simulink model "test"  (R2022a)
settings: Solver=VariableStepAuto  StartTime=0.0  StopTime=20  MaxStep=0.001  RelTol=1e-3
values from neighbouring files (symbols this model uses):
  SysMat = ss(Lmat)    [config.m]    (also in test_conf.m)
  SysVec = ss(Lvec)    [config.m]    (also in test_conf.m)
settings Model: Creator=Vvlad  LastModifiedBy=Vvlad

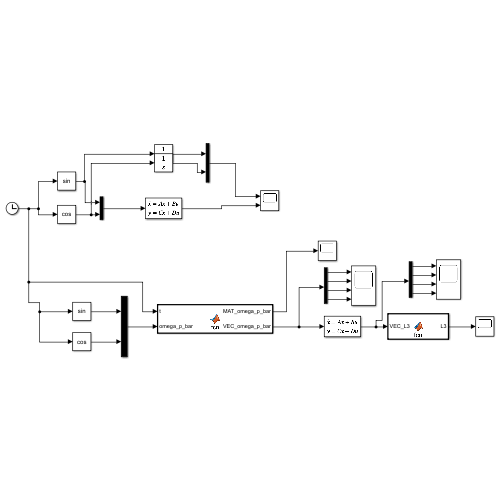
[thumbnail: Simulink's stored preview of the top-level diagram]
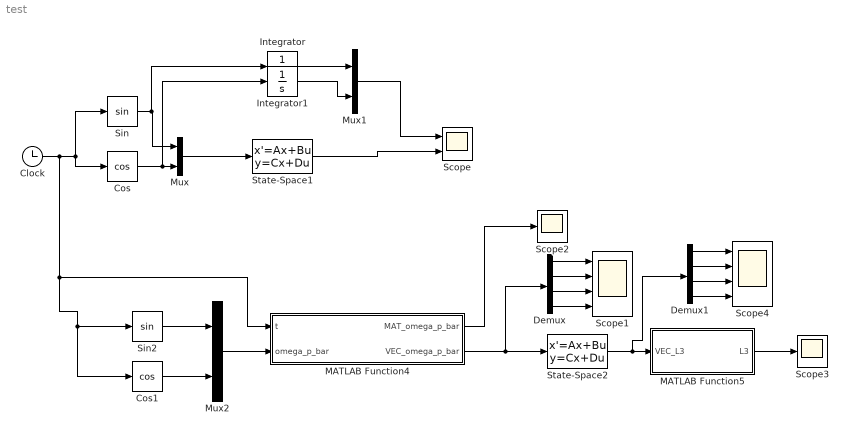
== system test ==
  Clock : Clock
  Cos : Trigonometry  Operator=cos
  Cos1 : Trigonometry  Operator=cos
  Demux : Demux
  Demux1 : Demux
  Integrator : Integrator
  Integrator1 : Integrator
  MATLAB Function4 : MATLAB Function  TreatAsAtomicUnit=on
  MATLAB Function5 : MATLAB Function  TreatAsAtomicUnit=on
  Mux : Mux  Inputs=2
  Mux1 : Mux  Inputs=2
  Mux2 : Mux  Inputs=2
  Scope : Scope  NumInputPorts=2
  Scope1 : Scope  NumInputPorts=4
  Scope2 : Scope
  Scope3 : Scope
  Scope4 : Scope  NumInputPorts=4
  Sin : Trigonometry
  Sin2 : Trigonometry
  State-Space1 : StateSpace  A=SysVec.A  B=SysVec.B  C=SysVec.C  D=SysVec.D  InitialCondition=0
  State-Space2 : StateSpace  A=SysMat.A  B=SysMat.B  C=SysMat.C  D=SysMat.D  InitialCondition=0
  wires:
  Sin/1 -> Integrator/1, Mux/1
  Clock/1 -> MATLAB Function4/1(t), Cos1/1, Sin2/1, Sin/1, Cos/1
  Cos/1 -> Integrator1/1, Mux/2
  Mux/1 -> State-Space1/1
  Integrator1/1 -> Mux1/2
  Integrator/1 -> Mux1/1
  State-Space1/1 -> Scope/2
  Mux1/1 -> Scope/1
  Cos1/1 -> Mux2/2
  Sin2/1 -> Mux2/1
  MATLAB Function4/2(VEC_omega_p_bar) -> Demux/1, State-Space2/1
  Demux/1 -> Scope1/1
  Demux/2 -> Scope1/2
  Demux/3 -> Scope1/3
  Demux/4 -> Scope1/4
  MATLAB Function4/1(MAT_omega_p_bar) -> Scope2/1
  Mux2/1 -> MATLAB Function4/2(omega_p_bar)
  Demux1/3 -> Scope4/3
  State-Space2/1 -> Demux1/1, MATLAB Function5/1(VEC_L3)
  Demux1/1 -> Scope4/1
  Demux1/2 -> Scope4/2
  Demux1/4 -> Scope4/4
  MATLAB Function5/1(L3) -> Scope3/1

== matlab function test/MATLAB Function5 ==
  data: VEC_L3 input; L3 output
function L3 = fcn(VEC_L3)
L3 = reshape(VEC_L3, 2,2);

== matlab function test/MATLAB Function4 ==
  data: t input; MAT_omega_p_bar output; omega_p_bar input; VEC_omega_p_bar output
function [MAT_omega_p_bar, VEC_omega_p_bar] = fcn(t, omega_p_bar)

MAT_omega_p_bar = omega_p_bar*omega_p_bar';
VEC_omega_p_bar = reshape(omega_p_bar*omega_p_bar', 4, 1);
VEC_omega_p_bar = [sin(t);
                   cos(t);
                   sin(t)*sin(t);
                   cos(t)*cos(t)];
